simulink model "zad2"  (R2022b)
settings: Solver=VariableStepAuto  StartTime=0.0  StopTime=100.0  MaxStep=0.1  RelTol=1e-3
libraries: slpidlib x2
settings Model: Creator=andre  LastModifiedBy=andre

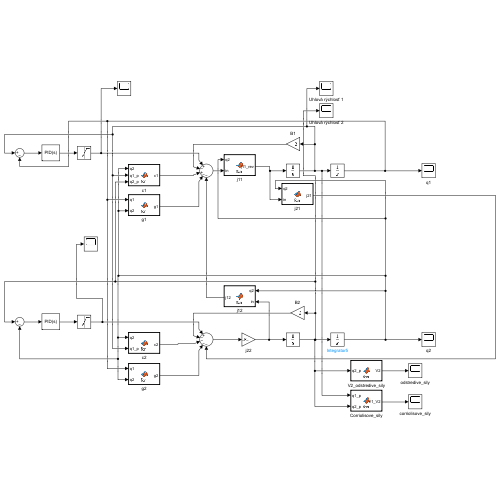
[thumbnail: Simulink's stored preview of the top-level diagram]
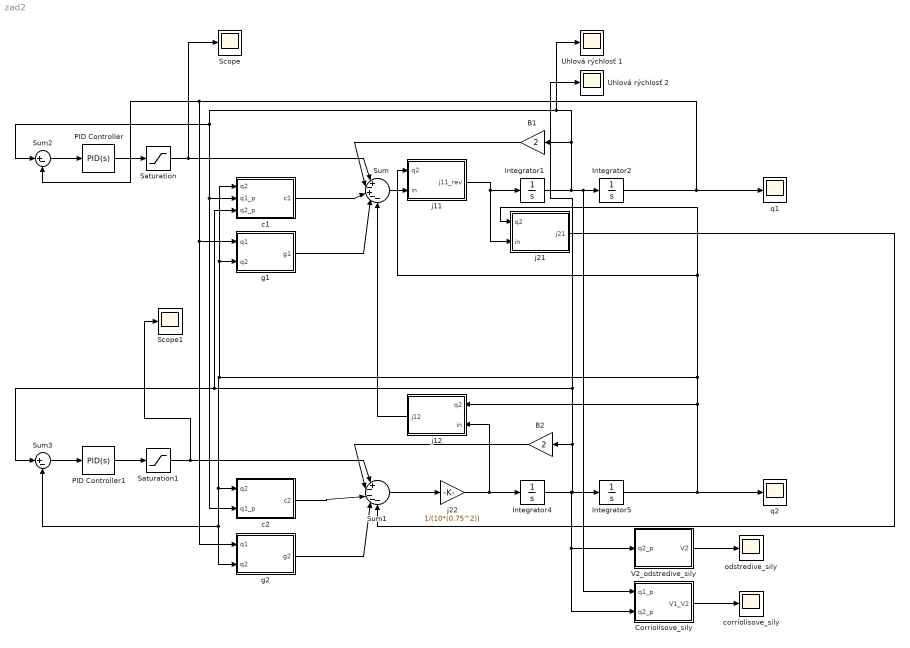
== system zad2 ==
  B1 : Gain  Gain=2
  B2 : Gain  Gain=2
  Corriolisove_sily : MATLAB Function  TreatAsAtomicUnit=on
  Integrator{1..2,4..5} (4 alike) : Integrator
  PID Controller : slpidlib/PID Controller  Controller=PID  Form=Parallel  TimeDomain=Continuous-time  UseExternalTs=off  SampleTime=-1  IntegratorMethod=Forward Euler  FilterMethod=Forward Euler  ControllerParametersSource=internal  P=1  I=1  UseKiTs=off  D=0  N=100  UseFilter=on  TunerSelectOption=Transfer Function Based (PID Tuner App)  InitialConditionSource=internal  InitialConditionForIntegrator=0  InitialConditionForFilter=0  DifferentiatorICPrevScaledInput=0  ExternalReset=none  TrackingMode=off  Kt=1  LimitOutput=off  SatLimitsSource=internal  UpperSaturationLimit=inf  LowerSaturationLimit=-inf  LinearizeAsGain=on  AntiWindupMode=none  Kb=1  LimitIntegrator=off  UpperIntegratorSaturationLimit=inf  LowerIntegratorSaturationLimit=-inf  POutMin=[]  POutMax=[]  IOutMin=[]  IOutMax=[]  DOutMin=[]  DOutMax=[]  NOutMin=[]  NOutMax=[]  SumOutMin=[]  SumOutMax=[]  SaturationOutMin=[]  SaturationOutMax=[]  PParamMin=[]  PParamMax=[]  IParamMin=[]  IParamMax=[]  DParamMin=[]  DParamMax=[]  NParamMin=[]  NParamMax=[]  KbParamMin=[]  KbParamMax=[]  KtParamMin=[]  KtParamMax=[]  KbOutMin=[]  KbOutMax=[]  KtOutMin=[]  KtOutMax=[]  IntegratorOutMin=[]  IntegratorOutMax=[]  FilterOutMin=[]  FilterOutMax=[]  SumI1OutMin=[]  SumI1OutMax=[]  SumI2OutMin=[]  SumI2OutMax=[]  SumI3OutMin=[]  SumI3OutMax=[]  SumI4OutMin=[]  SumI4OutMax=[]  SumDOutMin=[]  SumDOutMax=[]  DifferentiatorOutMin=[]  DifferentiatorOutMax=[]  FilterDiffOutCoefMin=[]  FilterDiffOutCoefMax=[]  ReciprocalOutMin=[]  ReciprocalOutMax=[]  SumDenOutMin=[]  SumDenOutMax=[]  SumNumOutMin=[]  SumNumOutMax=[]  DivideOutMin=[]  DivideOutMax=[]  UdiffTsProdOutMin=[]  UdiffTsProdOutMax=[]  NTsProdOutMin=[]  NTsProdOutMax=[]  UintegralTsProdOutMin=[]  UintegralTsProdOutMax=[]  UngainTsProdOutMin=[]  UngainTsProdOutMax=[]  ClampingZeroOutDataTypeStr=Inherit: Inherit via back propagation  ClampingZeroOutMin=[]  ClampingZeroOutMax=[]  FilterDenConstantOutDataTypeStr=Inherit: Inherit via back propagation  FilterDenConstantOutMin=[]  FilterDenConstantOutMax=[]  PCopyOutDataTypeStr=Inherit: Inherit via back propagation  PCopyOutMin=[]  PCopyOutMax=[]  NCopyOutDataTypeStr=Inherit: Inherit via back propagation  NCopyOutMin=[]  NCopyOutMax=[]  IntegratorContinuousStateAttributes=''  IntegratorStateMustResolveToSignalObject=off  IntegratorRTWStateStorageClass=Auto  FilterContinuousStateAttributes=''  FilterStateMustResolveToSignalObject=off  FilterRTWStateStorageClass=Auto  ParallelPVariant=InternalParameters  IdealPVariant=Disabled  IVariant=InternalParameters  DVariant=InternalParameters  IntegratorVariant=Continuous  SatVariant=Disabled  AWVariant=Passthrough  PCopyVariant=Disabled  TRVariant=Disabled  FdbkBlocksVariant=Forward  IdealPFdbkVariant=Disabled  SatFdbkVariant=Disabled  DerivativeFilterVariant=ContFilter  NVariant=InternalParameters  NCopyVariant=Disabled  FilterICVariant=InternalICsFilter  IntegratorICVariant=InternalICs  ExternalResetVariant=Disabled  TRSumVariant=Passthrough  SumFdbkVariant=Disabled  SumVariant=Sum_PID  TsampFilterVariant=InternalTs  TsampNgainVariant=Passthrough  TsampIntegralVariant=Passthrough  ExternalSaturationOutDataTypeStr=Inherit: Same as second input
  PID Controller1 : slpidlib/PID Controller  Controller=PID  Form=Parallel  TimeDomain=Continuous-time  UseExternalTs=off  SampleTime=-1  IntegratorMethod=Forward Euler  FilterMethod=Forward Euler  ControllerParametersSource=internal  P=1  I=1  UseKiTs=off  D=0  N=100  UseFilter=on  TunerSelectOption=Transfer Function Based (PID Tuner App)  InitialConditionSource=internal  InitialConditionForIntegrator=0  InitialConditionForFilter=0  DifferentiatorICPrevScaledInput=0  ExternalReset=none  TrackingMode=off  Kt=1  LimitOutput=off  SatLimitsSource=internal  UpperSaturationLimit=inf  LowerSaturationLimit=-inf  LinearizeAsGain=on  AntiWindupMode=none  Kb=1  LimitIntegrator=off  UpperIntegratorSaturationLimit=inf  LowerIntegratorSaturationLimit=-inf  POutMin=[]  POutMax=[]  IOutMin=[]  IOutMax=[]  DOutMin=[]  DOutMax=[]  NOutMin=[]  NOutMax=[]  SumOutMin=[]  SumOutMax=[]  SaturationOutMin=[]  SaturationOutMax=[]  PParamMin=[]  PParamMax=[]  IParamMin=[]  IParamMax=[]  DParamMin=[]  DParamMax=[]  NParamMin=[]  NParamMax=[]  KbParamMin=[]  KbParamMax=[]  KtParamMin=[]  KtParamMax=[]  KbOutMin=[]  KbOutMax=[]  KtOutMin=[]  KtOutMax=[]  IntegratorOutMin=[]  IntegratorOutMax=[]  FilterOutMin=[]  FilterOutMax=[]  SumI1OutMin=[]  SumI1OutMax=[]  SumI2OutMin=[]  SumI2OutMax=[]  SumI3OutMin=[]  SumI3OutMax=[]  SumI4OutMin=[]  SumI4OutMax=[]  SumDOutMin=[]  SumDOutMax=[]  DifferentiatorOutMin=[]  DifferentiatorOutMax=[]  FilterDiffOutCoefMin=[]  FilterDiffOutCoefMax=[]  ReciprocalOutMin=[]  ReciprocalOutMax=[]  SumDenOutMin=[]  SumDenOutMax=[]  SumNumOutMin=[]  SumNumOutMax=[]  DivideOutMin=[]  DivideOutMax=[]  UdiffTsProdOutMin=[]  UdiffTsProdOutMax=[]  NTsProdOutMin=[]  NTsProdOutMax=[]  UintegralTsProdOutMin=[]  UintegralTsProdOutMax=[]  UngainTsProdOutMin=[]  UngainTsProdOutMax=[]  ClampingZeroOutDataTypeStr=Inherit: Inherit via back propagation  ClampingZeroOutMin=[]  ClampingZeroOutMax=[]  FilterDenConstantOutDataTypeStr=Inherit: Inherit via back propagation  FilterDenConstantOutMin=[]  FilterDenConstantOutMax=[]  PCopyOutDataTypeStr=Inherit: Inherit via back propagation  PCopyOutMin=[]  PCopyOutMax=[]  NCopyOutDataTypeStr=Inherit: Inherit via back propagation  NCopyOutMin=[]  NCopyOutMax=[]  IntegratorContinuousStateAttributes=''  IntegratorStateMustResolveToSignalObject=off  IntegratorRTWStateStorageClass=Auto  FilterContinuousStateAttributes=''  FilterStateMustResolveToSignalObject=off  FilterRTWStateStorageClass=Auto  ParallelPVariant=InternalParameters  IdealPVariant=Disabled  IVariant=InternalParameters  DVariant=InternalParameters  IntegratorVariant=Continuous  SatVariant=Disabled  AWVariant=Passthrough  PCopyVariant=Disabled  TRVariant=Disabled  FdbkBlocksVariant=Forward  IdealPFdbkVariant=Disabled  SatFdbkVariant=Disabled  DerivativeFilterVariant=ContFilter  NVariant=InternalParameters  NCopyVariant=Disabled  FilterICVariant=InternalICsFilter  IntegratorICVariant=InternalICs  ExternalResetVariant=Disabled  TRSumVariant=Passthrough  SumFdbkVariant=Disabled  SumVariant=Sum_PID  TsampFilterVariant=InternalTs  TsampNgainVariant=Passthrough  TsampIntegralVariant=Passthrough  ExternalSaturationOutDataTypeStr=Inherit: Same as second input
  Saturation : Saturate  UpperLimit=80  LowerLimit=0
  Saturation1 : Saturate  UpperLimit=80  LowerLimit=0
  Scope : Scope
  Scope1 : Scope
  Sum : Sum  Inputs=|+-+--
  Sum1 : Sum  Inputs=|+----
  Sum2 : Sum  Inputs=|+-
  Sum3 : Sum  Inputs=|+-
  Uhlová rýchlosť 1 : Scope
  Uhlová rýchlosť 2 : Scope
  V2_odstredive_sily : MATLAB Function  TreatAsAtomicUnit=on
  c1 : MATLAB Function  TreatAsAtomicUnit=on
  c2 : MATLAB Function  TreatAsAtomicUnit=on
  corriolisove_sily : Scope
  g1 : MATLAB Function  TreatAsAtomicUnit=on
  g2 : MATLAB Function  TreatAsAtomicUnit=on
  j11 : MATLAB Function  TreatAsAtomicUnit=on
  j12 : MATLAB Function  TreatAsAtomicUnit=on
  j21 : MATLAB Function  TreatAsAtomicUnit=on
  j22 : Gain  Gain=1/(10*(0.75^2))
  odstredive_sily : Scope
  q1 : Scope
  q2 : Scope
  wires:
  Sum/1 -> j11/2(in)
  j11/1(j11_rev) -> j21/2(in), Integrator1/1
  Integrator1/1 -> B1/1, Uhlová rýchlosť 1/1, Sum2/1, c1/2(q1_p), c2/2(q1_p), Corriolisove_sily/1(q1_p), Integrator2/1
  Integrator2/1 -> Sum2/2, g2/1(q1), g1/1(q1), q1/1
  B1/1 -> Sum/2
  Sum1/1 -> j22/1
  j22/1 -> j12/2(in), Integrator4/1
  Integrator5/1 -> c1/1(q2), g1/2(q2), Sum3/2, g2/2(q2), c2/1(q2), j11/1(q2), j21/1(q2), j12/1(q2), q2/1
  B2/1 -> Sum1/2
  j12/1(j12) -> Sum/5
  j21/1(j21) -> Sum1/5
  c1/1(c1) -> Sum/3
  g1/1(g1) -> Sum/4
  c2/1(c2) -> Sum1/3
  g2/1(g2) -> Sum1/4
  Saturation/1 -> Scope/1, Sum/1
  Saturation1/1 -> Scope1/1, Sum1/1
  V2_odstredive_sily/1(V2) -> odstredive_sily/1
  Corriolisove_sily/1(V1_V2) -> corriolisove_sily/1
  Integrator4/1 -> Corriolisove_sily/2(q2_p), V2_odstredive_sily/1(q2_p), Uhlová rýchlosť 2/1, Sum3/1, c1/3(q2_p), B2/1, Integrator5/1
  PID Controller/1 -> Saturation/1
  PID Controller1/1 -> Saturation1/1
  Sum2/1 -> PID Controller/1
  Sum3/1 -> PID Controller1/1

== matlab function zad2/j11 ==
  data: q2 input; j11_rev output; in input
function j11_rev = fcn(q2, in)

j11_rev = in/(3*(10*(0.75^2)) + 2*10*(0.75^2)*cos(q2));

== matlab function zad2/j21 ==
  data: q2 input; j21 output; in input
function j21 = fcn(q2, in)

j21 = in*(10*(0.75^2)*cos(q2) + 10*(0.75^2));

== matlab function zad2/c1 ==
  data: q2 input; c1 output; q1_p input; q2_p input
function c1 = fcn(q2, q1_p, q2_p)

c1 = 10*(0.75^2)*q2_p*(2*q1_p + q2_p)*sin(q2);

== matlab function zad2/g1 ==
  data: q1 input; g1 output; q2 input
function g1 = fcn(q1, q2)

g1 = 10*9.81*0.75*cos(q1) + 10*9.81*(0.75*cos(q1) + 0.75*cos(q1 + q2));

== matlab function zad2/c2 ==
  data: q2 input; c2 output; q1_p input
function c2 = fcn(q2, q1_p)

c2 = 10*(0.75^2)*(q1_p^2)*sin(q2);

== matlab function zad2/g2 ==
  data: q1 input; g2 output; q2 input
function g2 = fcn(q1, q2)

g2 = 10*9.81*0.75*cos(q1 + q2);

== matlab function zad2/V2_odstredive_sily ==
  data: q2_p input; V2 output
function V2 = fcn(q2_p)

V2 = q2_p^2;

== matlab function zad2/Corriolisove_sily ==
  data: q1_p input; V1_V2 output; q2_p input
function V1_V2 = fcn(q1_p, q2_p)

V1_V2 = q1_p*q2_p;

== matlab function zad2/j12 ==
  data: q2 input; j12 output; in input
function j12 = fcn(q2, in)

j12 = in*(10*(0.75^2)*cos(q2) + 10*(0.75^2));
